simulink model "SEVEN_LEVEL_INV_WITH_Rl_LOAD - Copy"  (R2019a)
settings: Solver=ode23t  StartTime=0.0  StopTime=0.1  FixedStep=10e-8  MaxStep=1e-4  RelTol=1e-3
undefined symbols (not defined in the file): a1, a2, a3, Vdc
libraries: powerlib x50, simulink x3
settings Model: Creator=murra  LastModifiedBy=hp
settings DataIOCC: ReturnWorkspaceOutputs=off
settings DebuggingCC: SFMachineParentedDataDiag=error  ArithmeticOperatorsInVariantConditions=warning
settings CodeAppCC: StateflowObjectComments=on
settings SimscapeCC: SimscapeNormalizeSystem=off

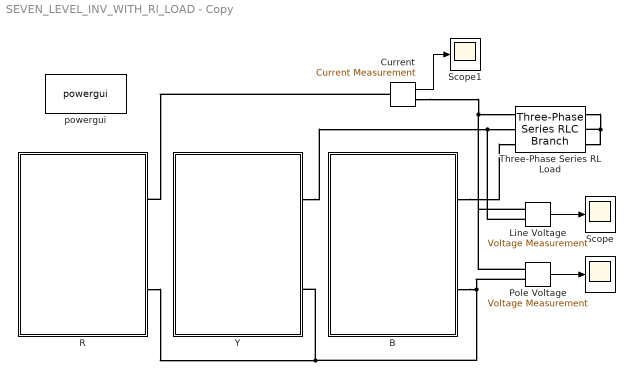
== system SEVEN_LEVEL_INV_WITH_Rl_LOAD - Copy ==
  " " : Scope
  B : Subsystem
  Current : powerlib/Measurements/Current Measurement  PhasorSimulation=off  OutputType=Complex  PSBequivalent=0
      settings: SourceProductName=Simscape Electrical
  Line Voltage : powerlib/Measurements/Voltage Measurement  PhasorSimulation=off  OutputType=Complex  PSBequivalent=0
      settings: SourceProductName=Simscape Electrical
  Pole Voltage : powerlib/Measurements/Voltage Measurement  PhasorSimulation=off  OutputType=Complex  PSBequivalent=0
      settings: SourceProductName=Simscape Electrical
  R : Subsystem
  Scope : Scope
  Scope1 : Scope
  Three-Phase Series RL Load : powerlib/Elements/Three-Phase Series RLC Branch  LConnTagsString=A|B|C  RConnTagsString=A|B|C  BranchType=RL  Resistance=100  Inductance=0.15  Capacitance=1e-6  Measurements=None
      settings: SourceProductName=Simscape Electrical
  Y : Subsystem
  powergui : powerlib/powergui  Priority=1  SimulationMode=Discrete  SampleTime=1e-6  frequency=60  Iterations=50  frequencyindice=0  Pbase=100e6  ErrMax=1e-4  UnitsV=kV  UnitsW=MW  buscounter=0  FunctionMessages=off  echomessages=off  EnableUseOfTLC=off  CurrentSourceSwitches=off  DisableSnubberDevices=off  DisableRonSwitches=off  DisableVfSwitches=off  DisplayEquations=off  AutomaticDiscreteSolvers=off  SolverType=Tustin/Backward Euler (TBE)  Interpol=off  ExternalGateDelay=off  methode=off  Ts=100  x0status=blocks  SPID=on  SwTol=0  HookPort=off  NonlinearTolerance=0  nMaxIteration=15  ContinueOnMaxIteration=off  RestoreLinks=warning  ResistiveCurrentMeasurement=off  Frange=[0:2:500]  Ylog=off  Xlog=on  ShowGrid=off  save=off  variable=ZData  structure=V  ZoomFFT=off  StartTime=0.02  cycles=2  DisplayStyle=2  fundamental=50  FreqAxis=off  MaxFrequency=1000  frequencyindicesteady=1  RmsSteady=1  display=off
      settings: SourceProductName=Simscape Electrical
  wires:
  Line Voltage/1 -> Scope/1
  Current/1 -> Scope1/1
  Pole Voltage/1 -> " "/1
  connections:
  Pole Voltage/LConn2 -- B/RConn2 -- R/RConn2 -- Y/RConn2
  Line Voltage/LConn1 -- Pole Voltage/LConn1 -- Current/RConn1 -- Three-Phase Series RL Load/LConn1
  Y/RConn1 -- Line Voltage/LConn2 -- Three-Phase Series RL Load/LConn2
  B/RConn1 -- Three-Phase Series RL Load/LConn3
  Current/LConn1 -- R/RConn1
  Three-Phase Series RL Load/RConn1 -- Three-Phase Series RL Load/RConn3 -- Three-Phase Series RL Load/RConn2

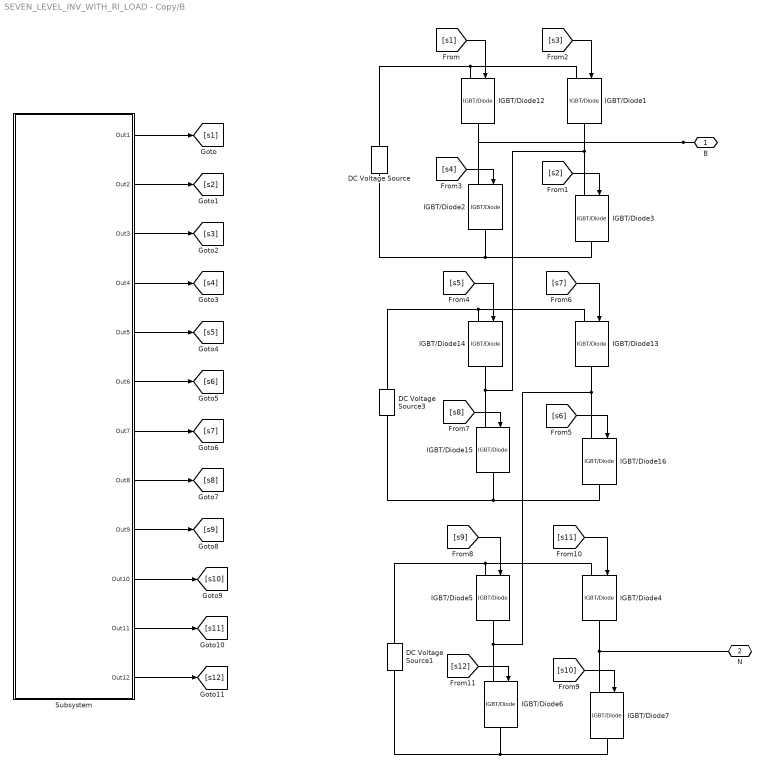
== system SEVEN_LEVEL_INV_WITH_Rl_LOAD - Copy/B ==
  DC Voltage Source : powerlib/Electrical Sources/DC Voltage Source  Amplitude=Vdc  Measurements=None
      settings: SourceProductName=Simscape Electrical
  DC Voltage Source1 : powerlib/Electrical Sources/DC Voltage Source  Amplitude=Vdc  Measurements=None
      settings: SourceProductName=Simscape Electrical
  DC Voltage Source3 : powerlib/Electrical Sources/DC Voltage Source  Amplitude=Vdc  Measurements=None
      settings: SourceProductName=Simscape Electrical
  IGBT/Diode{1..7,12..16} (12 alike) : powerlib/Power Electronics/IGBT//Diode  Ron=1e-3  Rs=1e5  Cs=inf  Measurements=off
      settings: SourceProductName=Simscape Electrical
  Subsystem : Subsystem
  B : PMIOPort  Side=Right
  N : PMIOPort  Port=2  Side=Right
  wires:
  [s3] -> IGBT/Diode1/1
  [s2] -> IGBT/Diode3/1
  [s1] -> IGBT/Diode12/1
  [s4] -> IGBT/Diode2/1
  [s12] -> IGBT/Diode6/1
  [s9] -> IGBT/Diode5/1
  [s10] -> IGBT/Diode7/1
  [s11] -> IGBT/Diode4/1
  [s7] -> IGBT/Diode13/1
  [s6] -> IGBT/Diode16/1
  [s5] -> IGBT/Diode14/1
  [s8] -> IGBT/Diode15/1
  Subsystem/5(Out5) -> [s5]
  Subsystem/3(Out3) -> [s3]
  Subsystem/6(Out6) -> [s6]
  Subsystem/1(Out1) -> [s1]
  Subsystem/11(Out11) -> [s11]
  Subsystem/4(Out4) -> [s4]
  Subsystem/8(Out8) -> [s8]
  Subsystem/7(Out7) -> [s7]
  Subsystem/9(Out9) -> [s9]
  Subsystem/10(Out10) -> [s10]
  Subsystem/12(Out12) -> [s12]
  Subsystem/2(Out2) -> [s2]
  connections:
  B/RConn1 -- IGBT/Diode2/LConn1 -- IGBT/Diode12/RConn1
  IGBT/Diode3/RConn1 -- DC Voltage Source/LConn1 -- IGBT/Diode2/RConn1
  IGBT/Diode15/LConn1 -- IGBT/Diode3/LConn1 -- IGBT/Diode1/RConn1 -- IGBT/Diode14/RConn1
  IGBT/Diode12/LConn1 -- DC Voltage Source/RConn1 -- IGBT/Diode1/LConn1
  DC Voltage Source1/LConn1 -- IGBT/Diode7/RConn1 -- IGBT/Diode6/RConn1
  DC Voltage Source1/RConn1 -- IGBT/Diode5/LConn1 -- IGBT/Diode4/LConn1
  IGBT/Diode4/RConn1 -- N/RConn1 -- IGBT/Diode7/LConn1
  IGBT/Diode16/RConn1 -- DC Voltage Source3/LConn1 -- IGBT/Diode15/RConn1
  IGBT/Diode14/LConn1 -- DC Voltage Source3/RConn1 -- IGBT/Diode13/LConn1
  IGBT/Diode6/LConn1 -- IGBT/Diode16/LConn1 -- IGBT/Diode13/RConn1 -- IGBT/Diode5/RConn1

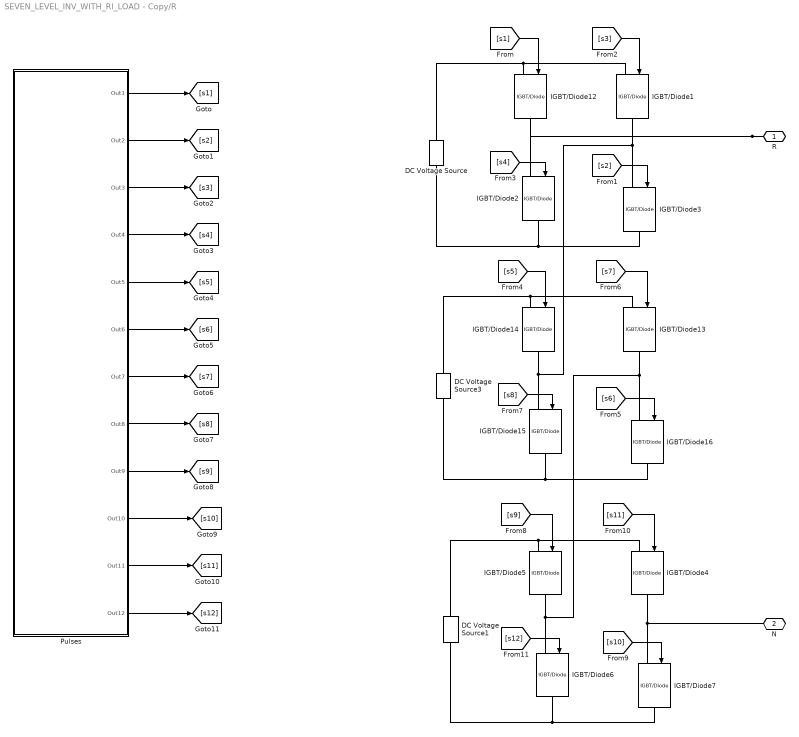
== system SEVEN_LEVEL_INV_WITH_Rl_LOAD - Copy/R ==
  DC Voltage Source : powerlib/Electrical Sources/DC Voltage Source  Amplitude=Vdc  Measurements=None
      settings: SourceProductName=Simscape Electrical
  DC Voltage Source1 : powerlib/Electrical Sources/DC Voltage Source  Amplitude=Vdc  Measurements=None
      settings: SourceProductName=Simscape Electrical
  DC Voltage Source3 : powerlib/Electrical Sources/DC Voltage Source  Amplitude=Vdc  Measurements=None
      settings: SourceProductName=Simscape Electrical
  IGBT/Diode{1..7,12..16} (12 alike) : powerlib/Power Electronics/IGBT//Diode  Ron=1e-3  Rs=1e5  Cs=inf  Measurements=off
      settings: SourceProductName=Simscape Electrical
  Pulses : Subsystem
  R : PMIOPort  Side=Right
  N : PMIOPort  Port=2  Side=Right
  wires:
  [s3] -> IGBT/Diode1/1
  [s2] -> IGBT/Diode3/1
  [s1] -> IGBT/Diode12/1
  [s4] -> IGBT/Diode2/1
  Pulses/1(Out1) -> [s1]
  Pulses/9(Out9) -> [s9]
  Pulses/2(Out2) -> [s2]
  Pulses/12(Out12) -> [s12]
  Pulses/4(Out4) -> [s4]
  Pulses/11(Out11) -> [s11]
  Pulses/10(Out10) -> [s10]
  Pulses/3(Out3) -> [s3]
  Pulses/5(Out5) -> [s5]
  [s12] -> IGBT/Diode6/1
  [s9] -> IGBT/Diode5/1
  [s10] -> IGBT/Diode7/1
  [s11] -> IGBT/Diode4/1
  [s7] -> IGBT/Diode13/1
  [s6] -> IGBT/Diode16/1
  [s5] -> IGBT/Diode14/1
  [s8] -> IGBT/Diode15/1
  Pulses/7(Out7) -> [s7]
  Pulses/6(Out6) -> [s6]
  Pulses/8(Out8) -> [s8]
  connections:
  R/RConn1 -- IGBT/Diode2/LConn1 -- IGBT/Diode12/RConn1
  IGBT/Diode3/RConn1 -- DC Voltage Source/LConn1 -- IGBT/Diode2/RConn1
  IGBT/Diode15/LConn1 -- IGBT/Diode3/LConn1 -- IGBT/Diode1/RConn1 -- IGBT/Diode14/RConn1
  IGBT/Diode12/LConn1 -- DC Voltage Source/RConn1 -- IGBT/Diode1/LConn1
  DC Voltage Source1/LConn1 -- IGBT/Diode7/RConn1 -- IGBT/Diode6/RConn1
  DC Voltage Source1/RConn1 -- IGBT/Diode5/LConn1 -- IGBT/Diode4/LConn1
  IGBT/Diode4/RConn1 -- N/RConn1 -- IGBT/Diode7/LConn1
  IGBT/Diode16/RConn1 -- DC Voltage Source3/LConn1 -- IGBT/Diode15/RConn1
  IGBT/Diode14/LConn1 -- DC Voltage Source3/RConn1 -- IGBT/Diode13/LConn1
  IGBT/Diode6/LConn1 -- IGBT/Diode16/LConn1 -- IGBT/Diode13/RConn1 -- IGBT/Diode5/RConn1

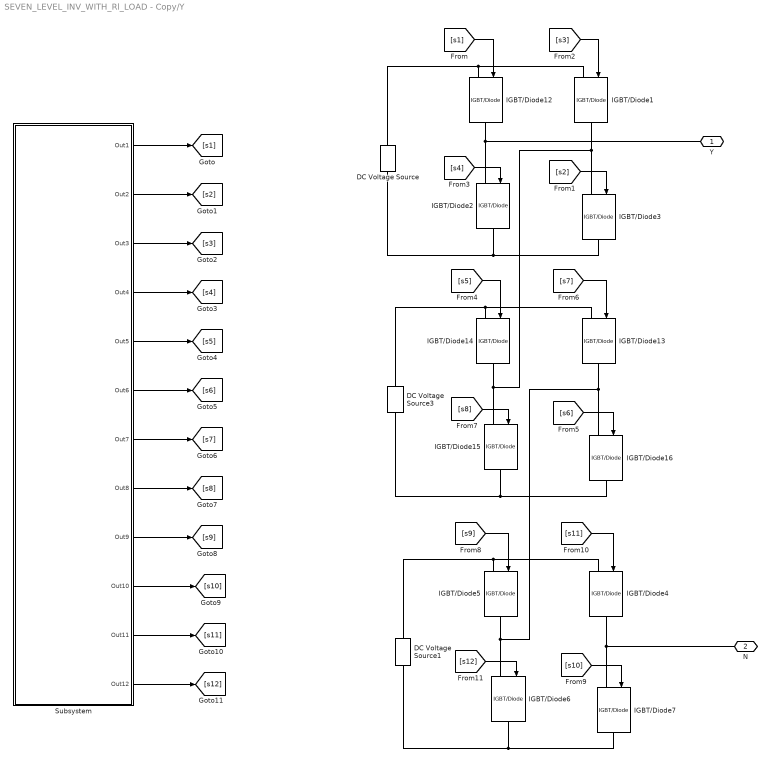
== system SEVEN_LEVEL_INV_WITH_Rl_LOAD - Copy/Y ==
  DC Voltage Source : powerlib/Electrical Sources/DC Voltage Source  Amplitude=Vdc  Measurements=None
      settings: SourceProductName=Simscape Electrical
  DC Voltage Source1 : powerlib/Electrical Sources/DC Voltage Source  Amplitude=Vdc  Measurements=None
      settings: SourceProductName=Simscape Electrical
  DC Voltage Source3 : powerlib/Electrical Sources/DC Voltage Source  Amplitude=Vdc  Measurements=None
      settings: SourceProductName=Simscape Electrical
  IGBT/Diode{1..7,12..16} (12 alike) : powerlib/Power Electronics/IGBT//Diode  Ron=1e-3  Rs=1e5  Cs=inf  Measurements=off
      settings: SourceProductName=Simscape Electrical
  Subsystem : Subsystem
  Y : PMIOPort  Side=Right
  N : PMIOPort  Port=2  Side=Right
  wires:
  [s8] -> IGBT/Diode15/1
  [s5] -> IGBT/Diode14/1
  [s6] -> IGBT/Diode16/1
  [s7] -> IGBT/Diode13/1
  [s11] -> IGBT/Diode4/1
  [s10] -> IGBT/Diode7/1
  [s9] -> IGBT/Diode5/1
  [s12] -> IGBT/Diode6/1
  [s4] -> IGBT/Diode2/1
  [s1] -> IGBT/Diode12/1
  [s2] -> IGBT/Diode3/1
  [s3] -> IGBT/Diode1/1
  Subsystem/5(Out5) -> [s5]
  Subsystem/3(Out3) -> [s3]
  Subsystem/6(Out6) -> [s6]
  Subsystem/1(Out1) -> [s1]
  Subsystem/11(Out11) -> [s11]
  Subsystem/4(Out4) -> [s4]
  Subsystem/8(Out8) -> [s8]
  Subsystem/7(Out7) -> [s7]
  Subsystem/9(Out9) -> [s9]
  Subsystem/10(Out10) -> [s10]
  Subsystem/12(Out12) -> [s12]
  Subsystem/2(Out2) -> [s2]
  connections:
  IGBT/Diode5/RConn1 -- IGBT/Diode13/RConn1 -- IGBT/Diode16/LConn1 -- IGBT/Diode6/LConn1
  IGBT/Diode13/LConn1 -- DC Voltage Source3/RConn1 -- IGBT/Diode14/LConn1
  IGBT/Diode15/RConn1 -- DC Voltage Source3/LConn1 -- IGBT/Diode16/RConn1
  IGBT/Diode7/LConn1 -- N/RConn1 -- IGBT/Diode4/RConn1
  IGBT/Diode4/LConn1 -- IGBT/Diode5/LConn1 -- DC Voltage Source1/RConn1
  IGBT/Diode6/RConn1 -- IGBT/Diode7/RConn1 -- DC Voltage Source1/LConn1
  IGBT/Diode1/LConn1 -- DC Voltage Source/RConn1 -- IGBT/Diode12/LConn1
  IGBT/Diode14/RConn1 -- IGBT/Diode1/RConn1 -- IGBT/Diode3/LConn1 -- IGBT/Diode15/LConn1
  IGBT/Diode2/RConn1 -- DC Voltage Source/LConn1 -- IGBT/Diode3/RConn1
  IGBT/Diode12/RConn1 -- IGBT/Diode2/LConn1 -- Y/RConn1

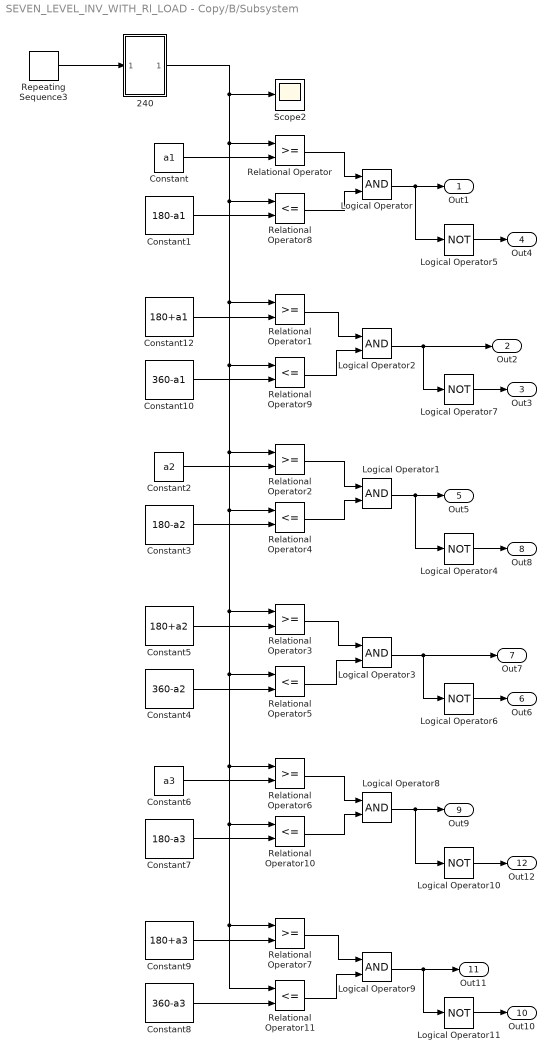
== system SEVEN_LEVEL_INV_WITH_Rl_LOAD - Copy/B/Subsystem ==
  240 : Subsystem
  Constant : Constant  Value=a1
  Constant1 : Constant  Value=180-a1
  Constant10 : Constant  Value=360-a1
  Constant12 : Constant  Value=180+a1
  Constant2 : Constant  Value=a2
  Constant3 : Constant  Value=180-a2
  Constant4 : Constant  Value=360-a2
  Constant5 : Constant  Value=180+a2
  Constant6 : Constant  Value=a3
  Constant7 : Constant  Value=180-a3
  Constant8 : Constant  Value=360-a3
  Constant9 : Constant  Value=180+a3
  Logical Operator{,1..3,8..9} (6 alike) : Logic  AllPortsSameDT=off  OutDataTypeStr=boolean
  Logical Operator{4..7,10..11} (6 alike) : Logic  Operator=NOT  AllPortsSameDT=off  OutDataTypeStr=boolean
  Relational Operator{,1..3,6..7} (6 alike) : RelationalOperator  OutDataTypeStr=boolean  RndMeth=Simplest
  Relational Operator{4..5,8..11} (6 alike) : RelationalOperator  Operator=<=  OutDataTypeStr=boolean  RndMeth=Simplest
  Repeating Sequence3 : simulink/Sources/Repeating Sequence  rep_seq_t=[0 0.02]  rep_seq_y=[0 360]
  Scope2 : Scope
  Out1 : Outport
  Out2 : Outport  Port=2
  Out3 : Outport  Port=3
  Out4 : Outport  Port=4
  Out5 : Outport  Port=5
  Out6 : Outport  Port=6
  Out7 : Outport  Port=7
  Out8 : Outport  Port=8
  Out9 : Outport  Port=9
  Out10 : Outport  Port=10
  Out11 : Outport  Port=11
  Out12 : Outport  Port=12
  wires:
  Logical Operator2/1 -> Logical Operator7/1, Out2/1
  Constant12/1 -> Relational Operator1/2
  Relational Operator8/1 -> Logical Operator/2
  Constant/1 -> Relational Operator/2
  Relational Operator/1 -> Logical Operator/1
  Constant1/1 -> Relational Operator8/2
  Logical Operator/1 -> Logical Operator5/1, Out1/1
  Relational Operator9/1 -> Logical Operator2/2
  Constant10/1 -> Relational Operator9/2
  Relational Operator1/1 -> Logical Operator2/1
  Logical Operator5/1 -> Out4/1
  Logical Operator7/1 -> Out3/1
  Logical Operator1/1 -> Out5/1, Logical Operator4/1
  Constant4/1 -> Relational Operator5/2
  Relational Operator5/1 -> Logical Operator3/2
  Constant3/1 -> Relational Operator4/2
  Relational Operator4/1 -> Logical Operator1/2
  Logical Operator4/1 -> Out8/1
  Relational Operator2/1 -> Logical Operator1/1
  Constant2/1 -> Relational Operator2/2
  Logical Operator3/1 -> Out7/1, Logical Operator6/1
  Logical Operator6/1 -> Out6/1
  Constant5/1 -> Relational Operator3/2
  Relational Operator3/1 -> Logical Operator3/1
  Logical Operator8/1 -> Out9/1, Logical Operator10/1
  Constant8/1 -> Relational Operator11/2
  Relational Operator11/1 -> Logical Operator9/2
  Constant7/1 -> Relational Operator10/2
  Relational Operator10/1 -> Logical Operator8/2
  Logical Operator10/1 -> Out12/1
  Relational Operator6/1 -> Logical Operator8/1
  Constant6/1 -> Relational Operator6/2
  Logical Operator9/1 -> Out11/1, Logical Operator11/1
  Logical Operator11/1 -> Out10/1
  Constant9/1 -> Relational Operator7/2
  Repeating Sequence3/1 -> 240/1(In1)
  Relational Operator7/1 -> Logical Operator9/1
  240/1(Out1) -> Relational Operator/1, Relational Operator8/1, Relational Operator2/1, Relational Operator4/1, Relational Operator6/1, Relational Operator10/1, Relational Operator11/1, Relational Operator7/1, Relational Operator5/1, Relational Operator3/1, Relational Operator9/1, Relational Operator1/1, Scope2/1

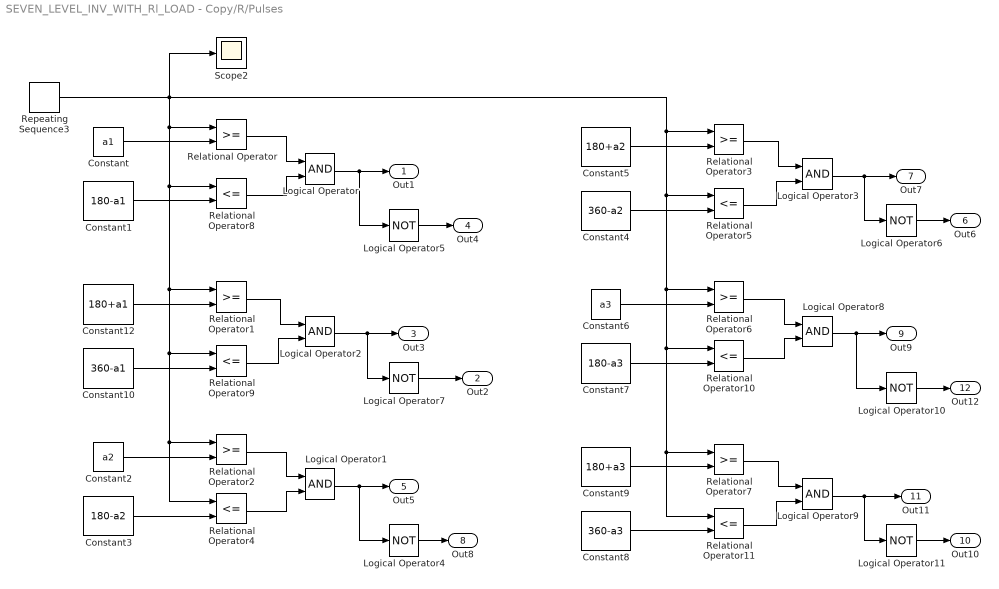
== system SEVEN_LEVEL_INV_WITH_Rl_LOAD - Copy/R/Pulses ==
  Constant : Constant  Value=a1
  Constant1 : Constant  Value=180-a1
  Constant10 : Constant  Value=360-a1
  Constant12 : Constant  Value=180+a1
  Constant2 : Constant  Value=a2
  Constant3 : Constant  Value=180-a2
  Constant4 : Constant  Value=360-a2
  Constant5 : Constant  Value=180+a2
  Constant6 : Constant  Value=a3
  Constant7 : Constant  Value=180-a3
  Constant8 : Constant  Value=360-a3
  Constant9 : Constant  Value=180+a3
  Logical Operator{,1..3,8..9} (6 alike) : Logic  AllPortsSameDT=off  OutDataTypeStr=boolean
  Logical Operator{4..7,10..11} (6 alike) : Logic  Operator=NOT  AllPortsSameDT=off  OutDataTypeStr=boolean
  Relational Operator{,1..3,6..7} (6 alike) : RelationalOperator  OutDataTypeStr=boolean  RndMeth=Simplest
  Relational Operator{4..5,8..11} (6 alike) : RelationalOperator  Operator=<=  OutDataTypeStr=boolean  RndMeth=Simplest
  Repeating Sequence3 : simulink/Sources/Repeating Sequence  rep_seq_t=[0 0.02]  rep_seq_y=[0 360]
  Scope2 : Scope
  Out1 : Outport
  Out2 : Outport  Port=2
  Out3 : Outport  Port=3
  Out4 : Outport  Port=4
  Out5 : Outport  Port=5
  Out6 : Outport  Port=6
  Out7 : Outport  Port=7
  Out8 : Outport  Port=8
  Out9 : Outport  Port=9
  Out10 : Outport  Port=10
  Out11 : Outport  Port=11
  Out12 : Outport  Port=12
  wires:
  Logical Operator2/1 -> Out3/1, Logical Operator7/1
  Constant12/1 -> Relational Operator1/2
  Relational Operator8/1 -> Logical Operator/2
  Constant/1 -> Relational Operator/2
  Relational Operator/1 -> Logical Operator/1
  Constant1/1 -> Relational Operator8/2
  Logical Operator/1 -> Logical Operator5/1, Out1/1
  Relational Operator9/1 -> Logical Operator2/2
  Constant10/1 -> Relational Operator9/2
  Relational Operator1/1 -> Logical Operator2/1
  Logical Operator5/1 -> Out4/1
  Logical Operator1/1 -> Out5/1, Logical Operator4/1
  Constant3/1 -> Relational Operator4/2
  Relational Operator4/1 -> Logical Operator1/2
  Relational Operator2/1 -> Logical Operator1/1
  Constant2/1 -> Relational Operator2/2
  Logical Operator7/1 -> Out2/1
  Constant6/1 -> Relational Operator6/2
  Logical Operator10/1 -> Out12/1
  Constant9/1 -> Relational Operator7/2
  Logical Operator9/1 -> Out11/1, Logical Operator11/1
  Logical Operator11/1 -> Out10/1
  Relational Operator10/1 -> Logical Operator8/2
  Constant5/1 -> Relational Operator3/2
  Relational Operator3/1 -> Logical Operator3/1
  Constant7/1 -> Relational Operator10/2
  Relational Operator7/1 -> Logical Operator9/1
  Repeating Sequence3/1 -> Relational Operator6/1, Relational Operator10/1, Relational Operator11/1, Relational Operator7/1, Relational Operator5/1, Relational Operator3/1, Scope2/1, Relational Operator/1, Relational Operator8/1, Relational Operator2/1, Relational Operator4/1, Relational Operator9/1, Relational Operator1/1
  Relational Operator6/1 -> Logical Operator8/1
  Constant8/1 -> Relational Operator11/2
  Constant4/1 -> Relational Operator5/2
  Logical Operator3/1 -> Out7/1, Logical Operator6/1
  Relational Operator5/1 -> Logical Operator3/2
  Logical Operator8/1 -> Out9/1, Logical Operator10/1
  Relational Operator11/1 -> Logical Operator9/2
  Logical Operator4/1 -> Out8/1
  Logical Operator6/1 -> Out6/1

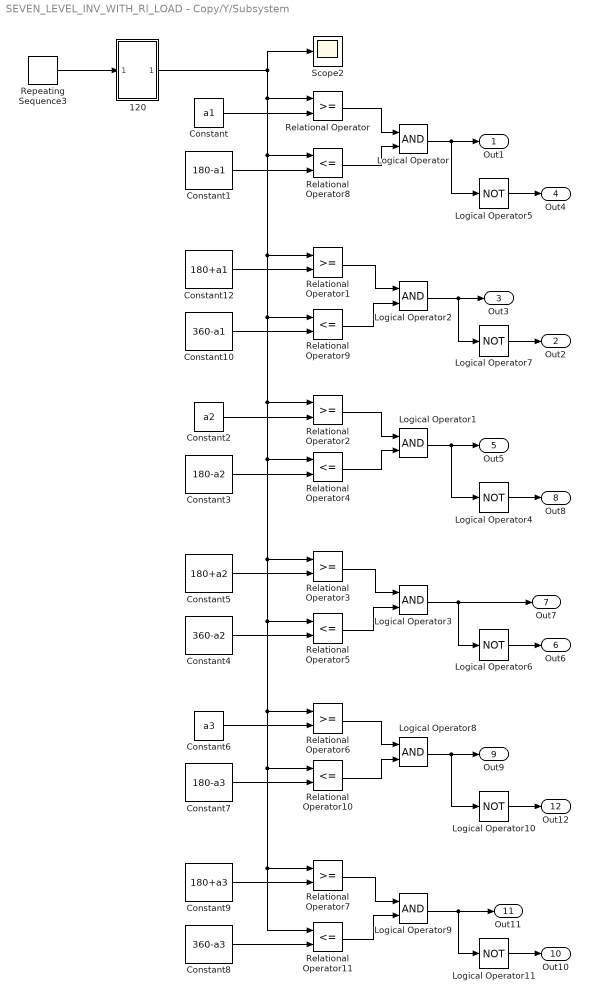
== system SEVEN_LEVEL_INV_WITH_Rl_LOAD - Copy/Y/Subsystem ==
  120 : Subsystem
  Constant : Constant  Value=a1
  Constant1 : Constant  Value=180-a1
  Constant10 : Constant  Value=360-a1
  Constant12 : Constant  Value=180+a1
  Constant2 : Constant  Value=a2
  Constant3 : Constant  Value=180-a2
  Constant4 : Constant  Value=360-a2
  Constant5 : Constant  Value=180+a2
  Constant6 : Constant  Value=a3
  Constant7 : Constant  Value=180-a3
  Constant8 : Constant  Value=360-a3
  Constant9 : Constant  Value=180+a3
  Logical Operator{,1..3,8..9} (6 alike) : Logic  AllPortsSameDT=off  OutDataTypeStr=boolean
  Logical Operator{4..7,10..11} (6 alike) : Logic  Operator=NOT  AllPortsSameDT=off  OutDataTypeStr=boolean
  Relational Operator{,1..3,6..7} (6 alike) : RelationalOperator  OutDataTypeStr=boolean  RndMeth=Simplest
  Relational Operator{4..5,8..11} (6 alike) : RelationalOperator  Operator=<=  OutDataTypeStr=boolean  RndMeth=Simplest
  Repeating Sequence3 : simulink/Sources/Repeating Sequence  rep_seq_t=[0 0.02]  rep_seq_y=[0 360]
  Scope2 : Scope
  Out1 : Outport
  Out2 : Outport  Port=2
  Out3 : Outport  Port=3
  Out4 : Outport  Port=4
  Out5 : Outport  Port=5
  Out6 : Outport  Port=6
  Out7 : Outport  Port=7
  Out8 : Outport  Port=8
  Out9 : Outport  Port=9
  Out10 : Outport  Port=10
  Out11 : Outport  Port=11
  Out12 : Outport  Port=12
  wires:
  Logical Operator2/1 -> Out3/1, Logical Operator7/1
  Constant12/1 -> Relational Operator1/2
  Relational Operator8/1 -> Logical Operator/2
  Constant/1 -> Relational Operator/2
  Relational Operator/1 -> Logical Operator/1
  Constant1/1 -> Relational Operator8/2
  Logical Operator/1 -> Logical Operator5/1, Out1/1
  Relational Operator9/1 -> Logical Operator2/2
  Constant10/1 -> Relational Operator9/2
  Relational Operator1/1 -> Logical Operator2/1
  Logical Operator5/1 -> Out4/1
  Logical Operator1/1 -> Out5/1, Logical Operator4/1
  Constant4/1 -> Relational Operator5/2
  Relational Operator5/1 -> Logical Operator3/2
  Constant3/1 -> Relational Operator4/2
  Relational Operator4/1 -> Logical Operator1/2
  Logical Operator4/1 -> Out8/1
  Relational Operator2/1 -> Logical Operator1/1
  Constant2/1 -> Relational Operator2/2
  Logical Operator3/1 -> Out7/1, Logical Operator6/1
  Logical Operator6/1 -> Out6/1
  Constant5/1 -> Relational Operator3/2
  Relational Operator3/1 -> Logical Operator3/1
  Logical Operator8/1 -> Out9/1, Logical Operator10/1
  Constant8/1 -> Relational Operator11/2
  Relational Operator11/1 -> Logical Operator9/2
  Constant7/1 -> Relational Operator10/2
  Relational Operator10/1 -> Logical Operator8/2
  Logical Operator10/1 -> Out12/1
  Relational Operator6/1 -> Logical Operator8/1
  Constant6/1 -> Relational Operator6/2
  Logical Operator9/1 -> Out11/1, Logical Operator11/1
  Logical Operator11/1 -> Out10/1
  Constant9/1 -> Relational Operator7/2
  Repeating Sequence3/1 -> 120/1(In1)
  Relational Operator7/1 -> Logical Operator9/1
  120/1(Out1) -> Scope2/1, Relational Operator/1, Relational Operator8/1, Relational Operator2/1, Relational Operator4/1, Relational Operator6/1, Relational Operator10/1, Relational Operator11/1, Relational Operator7/1, Relational Operator5/1, Relational Operator3/1, Relational Operator9/1, Relational Operator1/1
  Logical Operator7/1 -> Out2/1

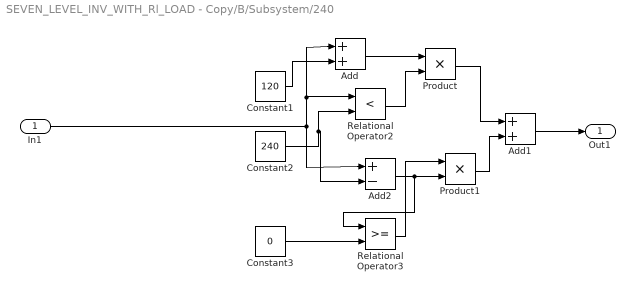
== system SEVEN_LEVEL_INV_WITH_Rl_LOAD - Copy/B/Subsystem/240 ==
  In1 : Inport
  Add : Sum  OutDataTypeStr=fixdt(1,15,0)
  Add1 : Sum  OutDataTypeStr=fixdt(1,15,0)
  Add2 : Sum  Inputs=+-  OutDataTypeStr=fixdt(1,15,0)
  Constant1 : Constant  Value=120  OutDataTypeStr=fixdt(0,14,0)  SampleTime=-1
  Constant2 : Constant  Value=240  OutDataTypeStr=fixdt(0,14,0)  SampleTime=-1
  Constant3 : Constant  Value=0  OutDataTypeStr=fixdt(0,14,0)  SampleTime=-1
  Product : Product
  Product1 : Product
  Relational Operator2 : RelationalOperator  Operator=<  OutDataTypeStr=fixdt(0,1,0)  RndMeth=Nearest
  Relational Operator3 : RelationalOperator  OutDataTypeStr=fixdt(0,1,0)  RndMeth=Nearest
  Out1 : Outport
  wires:
  Relational Operator2/1 -> Product/2
  Add2/1 -> Relational Operator3/1, Product1/2
  Add1/1 -> Out1/1
  Product1/1 -> Add1/2
  Product/1 -> Add1/1
  Constant2/1 -> Add2/2, Relational Operator2/2
  Constant3/1 -> Relational Operator3/2
  Relational Operator3/1 -> Product1/1
  Constant1/1 -> Add/2
  Add/1 -> Product/1
  In1/1 -> Add/1, Relational Operator2/1, Add2/1

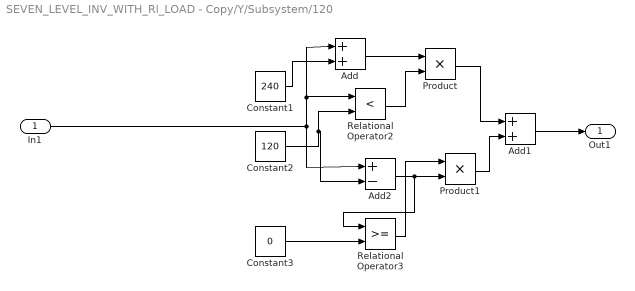
== system SEVEN_LEVEL_INV_WITH_Rl_LOAD - Copy/Y/Subsystem/120 ==
  In1 : Inport
  Add : Sum  OutDataTypeStr=fixdt(1,15,0)
  Add1 : Sum  OutDataTypeStr=fixdt(1,15,0)
  Add2 : Sum  Inputs=+-  OutDataTypeStr=fixdt(1,15,0)
  Constant1 : Constant  Value=240  OutDataTypeStr=fixdt(0,14,0)  SampleTime=-1
  Constant2 : Constant  Value=120  OutDataTypeStr=fixdt(0,14,0)  SampleTime=-1
  Constant3 : Constant  Value=0  OutDataTypeStr=fixdt(0,14,0)  SampleTime=-1
  Product : Product
  Product1 : Product
  Relational Operator2 : RelationalOperator  Operator=<  OutDataTypeStr=fixdt(0,1,0)  RndMeth=Nearest
  Relational Operator3 : RelationalOperator  OutDataTypeStr=fixdt(0,1,0)  RndMeth=Nearest
  Out1 : Outport
  wires:
  Relational Operator2/1 -> Product/2
  Add2/1 -> Relational Operator3/1, Product1/2
  Add1/1 -> Out1/1
  Product1/1 -> Add1/2
  Product/1 -> Add1/1
  Constant2/1 -> Add2/2, Relational Operator2/2
  Constant3/1 -> Relational Operator3/2
  Relational Operator3/1 -> Product1/1
  Constant1/1 -> Add/2
  Add/1 -> Product/1
  In1/1 -> Add/1, Relational Operator2/1, Add2/1
